simulink model "draft5"  (R2023a)
settings: Solver=VariableStepAuto  StartTime=0.0  StopTime=1  FixedStep=0.0001  MaxStep=0.2  RelTol=1e-3  AbsTol=1e-3  EnableMultiTasking=on
model workspace (MAT data in the model file):
  LeftAbdominalMuscleForce = -150
  LeftBackMuscleForce = -100
  LeftTransverseMucleForce1 = -100
  LeftTransverseMuscleForce2 = -100
  RightAbdominalMuscleForce = -150
  RightBackMuscleForce = -100
  RightTransverseMuscleForce1 = -150
  RightTransverseMuscleForce2 = -150
  c = 0.1
  k : Simulink.Parameter (value not decoded)
undefined symbols (not defined in the file or in its folder): X, Y, Z
libraries: nesl_utility x48, sm_lib x29, simulink_extras x3, checkpacklib x1
(part 3 of 3)

== matlab function draft5/L4/LB torque feedback L4/peacewise torque profile4 ==
  data: u input; torque output
function torque = T(u)
torque = 0;
if (u >= 15)
    torque= -0.0015*1*(57.295*15)^4 + 0.1326*(57.295*15)^3 -0.3477*(57.295*15)^2 + 0.499*(57.295*15);
 
elseif (u >= -15 && u<= 15)
    torque= -0.0015*(57.295*u)^4 + 0.1326*(57.295*u)^3 -0.3477*(57.295*u)^2 + 0.499*(57.295*u)   ;
    
elseif (u <= -15)
   torque= -0.0015*1*(57.295*-15)^4 + 0.1326*(57.295*-15)^3 -0.3477*(57.295*-15)^2 + 0.499*(57.295*-15);
end

== matlab function draft5/L4/AR torque feedback L4/peacewise torque profile5 ==
  data: u input; torque output
function torque = T(u)
torque = 0;
if (u >= 15)
    torque= -0.0015*1*(57.295*15)^4 + 0.1326*(57.295*15)^3 -0.3477*(57.295*15)^2 + 0.499*(57.295*15);
 
elseif (u >= -15 && u<= 15)
    torque= -0.0015*(57.295*u)^4 + 0.1326*(57.295*u)^3 -0.3477*(57.295*u)^2 + 0.499*(57.295*u)   ;
    
elseif (u <= -15)
   torque= -0.0015*1*(57.295*-15)^4 + 0.1326*(57.295*-15)^3 -0.3477*(57.295*-15)^2 + 0.499*(57.295*-15);
end

== matlab function draft5/L3/AR torque feedback L4/peacewise torque profile5 ==
  data: u input; torque output
function torque = T(u)
torque = 0;
if (u >= 15)
    torque= -0.0015*1*(57.295*15)^4 + 0.1326*(57.295*15)^3 -0.3477*(57.295*15)^2 + 0.499*(57.295*15);
 
elseif (u >= -15 && u<= 15)
    torque= -0.0015*(57.295*u)^4 + 0.1326*(57.295*u)^3 -0.3477*(57.295*u)^2 + 0.499*(57.295*u)   ;
    
elseif (u <= -15)
   torque= -0.0015*1*(57.295*-15)^4 + 0.1326*(57.295*-15)^3 -0.3477*(57.295*-15)^2 + 0.499*(57.295*-15);
end

== matlab function draft5/L3/FE torque feedback L4/peacewise torque profile1 ==
  data: u input; torque output
function torque = T(u)
torque = 0;
if (u >= 15)
    torque= -0.0015*1*(57.295*15)^4 + 0.1326*(57.295*15)^3 -0.3477*(57.295*15)^2 + 0.499*(57.295*15);
 
elseif (u >= -15 && u<= 15)
    torque= -0.0015*(57.295*u)^4 + 0.1326*(57.295*u)^3 -0.3477*(57.295*u)^2 + 0.499*(57.295*u)   ;
    
elseif (u <= -15)
   torque= -0.0015*1*(57.295*-15)^4 + 0.1326*(57.295*-15)^3 -0.3477*(57.295*-15)^2 + 0.499*(57.295*-15);
end

== matlab function draft5/L3/LB torque feedback L4/peacewise torque profile4 ==
  data: u input; torque output
function torque = T(u)
torque = 0;
if (u >= 15)
    torque= -0.0015*1*(57.295*15)^4 + 0.1326*(57.295*15)^3 -0.3477*(57.295*15)^2 + 0.499*(57.295*15);
 
elseif (u >= -15 && u<= 15)
    torque= -0.0015*(57.295*u)^4 + 0.1326*(57.295*u)^3 -0.3477*(57.295*u)^2 + 0.499*(57.295*u)   ;
    
elseif (u <= -15)
   torque= -0.0015*1*(57.295*-15)^4 + 0.1326*(57.295*-15)^3 -0.3477*(57.295*-15)^2 + 0.499*(57.295*-15);
end

== matlab function draft5/L4/FE torque feedback L4/peacewise torque profile1 ==
  data: u input; torque output
function torque = T(u)
torque = 0;
if (u >= 15)
    torque= -0.0015*1*(57.295*15)^4 + 0.1326*(57.295*15)^3 -0.3477*(57.295*15)^2 + 0.499*(57.295*15);
 
elseif (u >= -15 && u<= 15)
    torque= -0.0015*(57.295*u)^4 + 0.1326*(57.295*u)^3 -0.3477*(57.295*u)^2 + 0.499*(57.295*u)   ;
    
elseif (u <= -15)
   torque= -0.0015*1*(57.295*-15)^4 + 0.1326*(57.295*-15)^3 -0.3477*(57.295*-15)^2 + 0.499*(57.295*-15);
end

== matlab function draft5/L2/AR torque feedback L4/peacewise torque profile5 ==
  data: u input; torque output
function torque = T(u)
torque = 0;
if (u >= 15)
    torque= -0.0015*1*(57.295*15)^4 + 0.1326*(57.295*15)^3 -0.3477*(57.295*15)^2 + 0.499*(57.295*15);
 
elseif (u >= -15 && u<= 15)
    torque= -0.0015*(57.295*u)^4 + 0.1326*(57.295*u)^3 -0.3477*(57.295*u)^2 + 0.499*(57.295*u)   ;
    
elseif (u <= -15)
   torque= -0.0015*1*(57.295*-15)^4 + 0.1326*(57.295*-15)^3 -0.3477*(57.295*-15)^2 + 0.499*(57.295*-15);
end

== matlab function draft5/L2/FE torque feedback L4/peacewise torque profile1 ==
  data: u input; torque output
function torque = T(u)
torque = 0;
if (u >= 15)
    torque= -0.0015*1*(57.295*15)^4 + 0.1326*(57.295*15)^3 -0.3477*(57.295*15)^2 + 0.499*(57.295*15);
 
elseif (u >= -15 && u<= 15)
    torque= -0.0015*(57.295*u)^4 + 0.1326*(57.295*u)^3 -0.3477*(57.295*u)^2 + 0.499*(57.295*u)   ;
    
elseif (u <= -15)
   torque= -0.0015*1*(57.295*-15)^4 + 0.1326*(57.295*-15)^3 -0.3477*(57.295*-15)^2 + 0.499*(57.295*-15);
end

== matlab function draft5/L2/LB torque feedback L4/peacewise torque profile4 ==
  data: u input; torque output
function torque = T(u)
torque = 0;
if (u >= 15)
    torque= -0.0015*1*(57.295*15)^4 + 0.1326*(57.295*15)^3 -0.3477*(57.295*15)^2 + 0.499*(57.295*15);
 
elseif (u >= -15 && u<= 15)
    torque= -0.0015*(57.295*u)^4 + 0.1326*(57.295*u)^3 -0.3477*(57.295*u)^2 + 0.499*(57.295*u)   ;
    
elseif (u <= -15)
   torque= -0.0015*1*(57.295*-15)^4 + 0.1326*(57.295*-15)^3 -0.3477*(57.295*-15)^2 + 0.499*(57.295*-15);
end

== matlab function draft5/L1/AR torque feedback L4/peacewise torque profile5 ==
  data: u input; torque output
function torque = T(u)
torque = 0;
if (u >= 15)
    torque= -0.0015*1*(57.295*15)^4 + 0.1326*(57.295*15)^3 -0.3477*(57.295*15)^2 + 0.499*(57.295*15);
 
elseif (u >= -15 && u<= 15)
    torque= -0.0015*(57.295*u)^4 + 0.1326*(57.295*u)^3 -0.3477*(57.295*u)^2 + 0.499*(57.295*u)   ;
    
elseif (u <= -15)
   torque= -0.0015*1*(57.295*-15)^4 + 0.1326*(57.295*-15)^3 -0.3477*(57.295*-15)^2 + 0.499*(57.295*-15);
end

== matlab function draft5/L1/FE torque feedback L4/peacewise torque profile1 ==
  data: u input; torque output
function torque = T(u)
torque = 0;
if (u >= 15)
    torque= -0.0015*1*(57.295*15)^4 + 0.1326*(57.295*15)^3 -0.3477*(57.295*15)^2 + 0.499*(57.295*15);
 
elseif (u >= -15 && u<= 15)
    torque= -0.0015*(57.295*u)^4 + 0.1326*(57.295*u)^3 -0.3477*(57.295*u)^2 + 0.499*(57.295*u)   ;
    
elseif (u <= -15)
   torque= -0.0015*1*(57.295*-15)^4 + 0.1326*(57.295*-15)^3 -0.3477*(57.295*-15)^2 + 0.499*(57.295*-15);
end
